simulink model "Modulation_pure"  (Simulink 6.5)
settings: Solver=ode45  StartTime=0.0  StopTime=15.0  RelTol=1e-3
libraries: simulink x2
settings Model: DataTypeOverride=TrueDoubles  MinMaxOverflowLogging=ForceOff  Creator=arekg  LastModifiedBy=arekg
settings DataIOCC: SignalLoggingName=sigsOut
settings OptimizationCC: InlineInvariantSignals=on
settings DebuggingCC: SolverPrmCheckMsg=none  MultiTaskDSMMsg=warning  MultiTaskCondExecSysMsg=none  StrictBusMsg=None
settings HardwareCC: TargetUnknown=on
settings RTWCC: IncludeERTFirstTime=on
settings GRTTargetCC: ModelReferenceCompliant=off  MatFileLogging=off

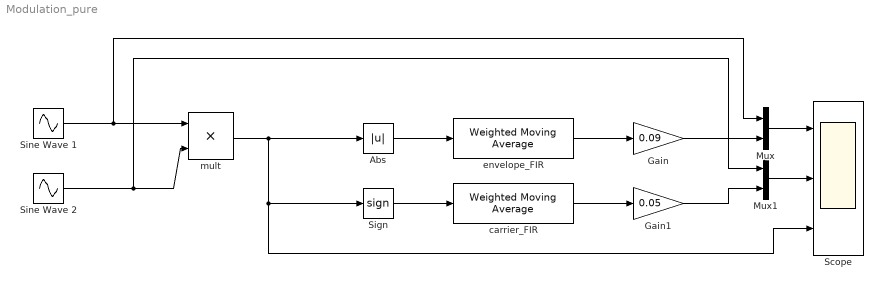
== system Modulation_pure ==
  Abs : Abs  SaturateOnIntegerOverflow=on  ZeroCross=off  SampleTime=1/20
  Gain : Gain  Gain=0.09  SampleTime=1/20
  Gain1 : Gain  Gain=0.05  SampleTime=1/20
  Mux : Mux  Inputs=2
  Mux1 : Mux  Inputs=2
  Scope : Scope  NumInputPorts=3
      settings: TimeRange=15  YMin=0~-1.5~-40  YMax=40~1.5~40
  Sign : Signum  ZeroCross=off  SampleTime=1/20
  Sine Wave 1 : Sin  Amplitude=18  Bias=20  Frequency=0.2*(2*pi)  Phase=pi/1.3  SampleTime=1/20
  Sine Wave 2 : Sin  Amplitude=0.9  Frequency=1.18*(2*pi)  Phase=pi  SampleTime=1/20
  carrier_FIR : simulink/Discrete/Weighted Moving Average  mgainval=[0.5982 1.421 2.3924 3.41 4.3567 3.41 2.3924 1.421 0.5982]  vinit=0.0  samptime=1/20  GainDataTypeScalingMode=Specify via dialog  GainDataType=sfix( 16 )  MatRadixGroup=Best Precision: Matrix-wise  GainScaling=2^-12  OutputDataTypeScalingMode=Specify via dialog  OutDataType=sfix(16)  OutScaling=2^-10  DoSatur=off
  envelope_FIR : simulink/Discrete/Weighted Moving Average  mgainval=[2.2649 1.7647 2.1936 2.4839 2.5857 2.4839 2.1936 1.7647 2.2649]  vinit=0.0  samptime=1/20  GainDataTypeScalingMode=Specify via dialog  GainDataType=sfix( 16 )  MatRadixGroup=Best Precision: Matrix-wise  GainScaling=2^-13  OutputDataTypeScalingMode=Specify via dialog  OutDataType=sfix(16)  OutScaling=2^-10  DoSatur=off
  mult : Product  OutDataTypeMode=double  SampleTime=1/20  SaturateOnIntegerOverflow=on  RndMeth=Zero
  wires:
  Sine Wave 1/1 -> Mux/1, mult/1
  Sine Wave 2/1 -> Mux1/1, mult/2
  mult/1 -> Scope/3, Sign/1, Abs/1
  Mux/1 -> Scope/1
  envelope_FIR/1 -> Gain/1
  Mux1/1 -> Scope/2
  carrier_FIR/1 -> Gain1/1
  Abs/1 -> envelope_FIR/1
  Sign/1 -> carrier_FIR/1
  Gain1/1 -> Mux1/2
  Gain/1 -> Mux/2
